simulink model "hw_interface_uart_data_receiver"  (R2023b)
settings: Solver=FixedStepAuto  StartTime=0.0  StopTime=inf  FixedStep=0.0005  RelTol=1e-3
undefined symbols (not defined in the file): LF
libraries: instrumentseriallib x2, embeddedblockslib x1, simulink_extras x1
settings Model: Creator=kiraa  LastModifiedBy=kiraa

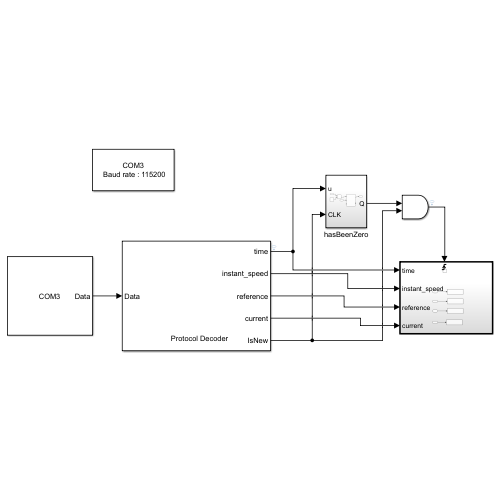
[thumbnail: Simulink's stored preview of the top-level diagram]
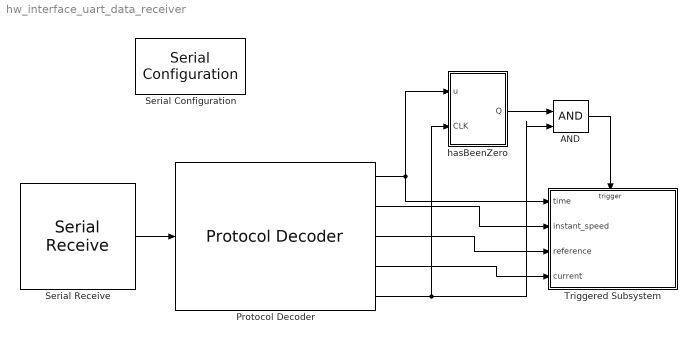
== system hw_interface_uart_data_receiver ==
  AND : Logic  IconShape=distinctive  AllPortsSameDT=off  OutDataTypeStr=boolean
  Protocol Decoder : embeddedblockslib/Protocol Decoder  IsParseCSV=off  Header='$'  FieldTable={ 'time', '1', 'double', 'Little endian'; 'instant_speed', '1', 'double', 'Little endian'; 'reference', '1', 'double', 'Little endian'; 'current', '1', 'double', 'Little endian' }  IsVariableSizeLastField=off  MaxVariableSizeFieldLength=[]  IsChecksumRequired=off  ChecksumAlgorithm=XOR of bytes  ChecksumSize=[]  TerminatorOption=LF ('\n')  CustomTerminatorVal=[]  IsInputLengthAvailable=off
      settings: LibrarySourceBlock=nucleoutilitieslib/Protocol Decoder
  Serial Configuration : instrumentseriallib/Serial Configuration  Priority=-200000  PortSel=COM3  Port=COM3  ComPort=COM3  BaudRate=115200  DataBits=8  Parity=none  StopBits=1  ByteOrder=little-endian  FlowControl=none  Timeout=10  SimulateUsing=Interpreted execution  BlockInModel=on  aMode=1
      settings: LibrarySourceBlock=embeddedtargetslib/Host Communication/Serial Configuration
  Serial Receive : instrumentseriallib/Serial Receive  Priority=1  PortSel=COM3  Port=COM3  ComPort=COM3  DataType=uint8  SaveDataType=uint8  ToggleHeader=off  Header=36  DataSize=[4]  ToggleTerminator=off  Terminator=LF ('\n')  CustomTerminator=[]  InputFormat=Column major  ToggleDataSize=on  EnableBlockingMode=on  ActionDataUnavailable=Output last received value  ActionWhenDataUnavailable=Output last received value  CustomValue=0  SampleTime=-1  SimulateUsing=Interpreted execution  BlockInModel=on  aMode=1
      settings: LibrarySourceBlock=embeddedtargetslib/Host Communication/Serial Receive
  Triggered Subsystem : Subsystem  TreatAsAtomicUnit=on
  hasBeenZero : Subsystem
  wires:
  Serial Receive/1 -> Protocol Decoder/1
  Protocol Decoder/1 -> Triggered Subsystem/1(time), hasBeenZero/1(u)
  Protocol Decoder/3 -> Triggered Subsystem/3(reference)
  Protocol Decoder/4 -> Triggered Subsystem/4(current)
  Protocol Decoder/5 -> AND/2, hasBeenZero/2(CLK)
  hasBeenZero/1(Q) -> AND/1
  AND/1 -> Triggered Subsystem/Trigger
  Protocol Decoder/2 -> Triggered Subsystem/2(instant_speed)

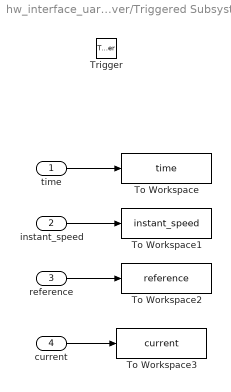
== system hw_interface_uart_data_receiver/Triggered Subsystem ==
  time : Inport  PortDimensions=1
  instant_speed : Inport  Port=2  PortDimensions=1
  reference : Inport  Port=3  PortDimensions=1
  current : Inport  Port=4  PortDimensions=1
  Trigger : TriggerPort  VariantControl=(inherit)  OutputDataType=int8
  To Workspace : ToWorkspace  VariableName=time  SaveFormat=Timeseries  SampleTime=-1
  To Workspace1 : ToWorkspace  VariableName=instant_speed  SaveFormat=Timeseries  SampleTime=-1
  To Workspace2 : ToWorkspace  VariableName=reference  SaveFormat=Timeseries  SampleTime=-1
  To Workspace3 : ToWorkspace  VariableName=current  SaveFormat=Timeseries  SampleTime=-1
  wires:
  instant_speed/1 -> To Workspace1/1
  reference/1 -> To Workspace2/1
  time/1 -> To Workspace/1
  current/1 -> To Workspace3/1

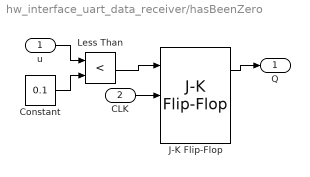
== system hw_interface_uart_data_receiver/hasBeenZero ==
  u : Inport
  CLK : Inport  Port=2
  Constant : Constant  Value=0.1
  J-K Flip-Flop : simulink_extras/Flip Flops/J-K Flip-Flop  initial_condition=0
  Less Than : RelationalOperator  Operator=<  OutDataTypeStr=boolean  RndMeth=Simplest  InputSameDT=off
  Q : Outport
  wires:
  u/1 -> Less Than/1
  Less Than/1 -> J-K Flip-Flop/1
  J-K Flip-Flop/1 -> Q/1
  CLK/1 -> J-K Flip-Flop/2
  Constant/1 -> Less Than/2
